simulink model "TSR_Scenario_001_cs"  (R2014b)
settings: Solver=ode5  SolverMode=SingleTasking  StartTime=0.0  StopTime=inf  FixedStep=1/100  RelTol=1e-3
PreLoadFcn:
  | mbxruntime.callbacks.PreLoadFcn(bdroot);
  | check_NUTS_defined;
  | 
  | assignin('base',['model_closed_' bdroot],false);
  | 
  | addpath('../includes_TSR/includes_TSR');
  | 
  | switch version('-release')
  | case {'2010a', '2010b', '2011a'}
  | addpath('../includes_TSR/ML2010b');
  | otherwise
  | addpath('../includes_TSR/ML2011b');
  | end
PostLoadFcn:
  | mbxruntime.callbacks.PostLoadFcn(bdroot);
InitFcn:
  | mbxruntime.callbacks.InitFcn(bdroot);
StartFcn:
  | mbxruntime.callbacks.StartFcn(bdroot);
StopFcn:
  | mbxruntime.callbacks.StopFcn(bdroot);
model workspace: external: MAT-File .\TSR_Scenario_001_cs_hws.mat (data not in the file)
undefined symbols (not defined in the file or in its folder): InitImageOutputDir, mbxruntime, OrientationPitch, OrientationRoll, PositionX, PositionY, PositionZ, tabledata, warningInitialVelocity, x0
undefined symbols (not defined in the file): SteeringColumn, SteeringWheel, TSR_Scenario_001_cs_0469e6db089af631, TSR_Scenario_001_cs_0511100212e7bc8e, TSR_Scenario_001_cs_0e7e9ae969427aac, TSR_Scenario_001_cs_1093386e49c2fe1f, TSR_Scenario_001_cs_112063adae8cf595, TSR_Scenario_001_cs_20f00d93cd5331c2, TSR_Scenario_001_cs_23e3512474fbfadc, TSR_Scenario_001_cs_366523e1554c6bf4, TSR_Scenario_001_cs_37bce4982c67337a, TSR_Scenario_001_cs_44e6164a5df50f45, TSR_Scenario_001_cs_4963ce12e7ff3247, TSR_Scenario_001_cs_4b3e01fa729ce73a, TSR_Scenario_001_cs_519c34727ce9f069, TSR_Scenario_001_cs_5b66ab60038399a1, TSR_Scenario_001_cs_5baa165dfa1afdcb, TSR_Scenario_001_cs_5f993ce39fa6372c, TSR_Scenario_001_cs_613fdf28e3ff7437, TSR_Scenario_001_cs_67b1406af835d622, TSR_Scenario_001_cs_6ad990c290286b94, TSR_Scenario_001_cs_6c412b69295984e1, TSR_Scenario_001_cs_6d4c0c06b1585ef3, TSR_Scenario_001_cs_6dd019d071bf1235, TSR_Scenario_001_cs_6e9f5883f1a78533, TSR_Scenario_001_cs_80f7223d9ac35404, TSR_Scenario_001_cs_8562b82d3c89ae57, TSR_Scenario_001_cs_8a3a0181ab0babfe, TSR_Scenario_001_cs_8c997348ce80deaf, TSR_Scenario_001_cs_925bd6a073d9fe25, TSR_Scenario_001_cs_961436216add6114, TSR_Scenario_001_cs_991a7959256b2c84, TSR_Scenario_001_cs_9a95ce2c2e753616, TSR_Scenario_001_cs_a98aa9562e8552a9, TSR_Scenario_001_cs_ab44ae81dbfb58cd, TSR_Scenario_001_cs_Actros_2541_2_Path_pathUniqueID, TSR_Scenario_001_cs_ae74836ade6bff5a, TSR_Scenario_001_cs_Audi_A8_1_Dynamics_Simple_initialPitch, TSR_Scenario_001_cs_Audi_A8_1_Dynamics_Simple_initialRoll, TSR_Scenario_001_cs_Audi_A8_1_Dynamics_Simple_initialX, TSR_Scenario_001_cs_Audi_A8_1_Dynamics_Simple_initialY, TSR_Scenario_001_cs_Audi_A8_1_Dynamics_Simple_initialYaw, TSR_Scenario_001_cs_Audi_A8_1_Dynamics_Simple_initialZ, TSR_Scenario_001_cs_Audi_A8_2_Path_pathUniqueID, TSR_Scenario_001_cs_Audi_A8_2_SpeedProfile_speedProfileUniqueID, TSR_Scenario_001_cs_b2eca4eb2fce349a, TSR_Scenario_001_cs_b7bac209c1f2549f, TSR_Scenario_001_cs_bf3dccb66d3255a4, TSR_Scenario_001_cs_bf4c1a5315e3f716, TSR_Scenario_001_cs_BMW_Z3_1_Path_pathUniqueID, TSR_Scenario_001_cs_BMW_Z3_1_SpeedProfile_speedProfileUniqueID, TSR_Scenario_001_cs_BMW_Z3_2_Path_pathUniqueID, TSR_Scenario_001_cs_BMW_Z3_2_SpeedProfile_speedProfileUniqueID, TSR_Scenario_001_cs_c4c8fc4bdece03a9, TSR_Scenario_001_cs_c964c86aa54ad92e, TSR_Scenario_001_cs_cb64d1ef85329755, TSR_Scenario_001_cs_Citroen_C3_1_Path_pathUniqueID, TSR_Scenario_001_cs_Citroen_C3_2_Path_pathUniqueID, TSR_Scenario_001_cs_Citroen_C3_3_Path_pathUniqueID, TSR_Scenario_001_cs_Citroen_C3_4_Path_pathUniqueID ... (+25)
libraries: simulink x21, PreScanSimulinkLibrary x17, simulink_extras x13
(part 3 of 30)

== system TSR_Scenario_001_cs/Audi_A8_1_Indicator_front_right ==
  Audi_A8_1_Indicator_front_right : Inport  Tag=inport/IndicatorFR  OutDataTypeStr=Bus: PRESCAN_VISULIGHTACTUATOR_DATA  SampleTime=1/100  BusOutputAsStruct=on
  Actuator : S-Function  FunctionName=sfun_VisuLightActuator  Parameters=mbxruntime.parameters.convert(UniqueID), mbxruntime.parameters.convert(LightName), mbxruntime.parameters.convert(PivotName), mbxruntime.parameters.convert(TextureResources), mbxruntime.parameters.convert(ColorsObjectName), mbxruntime.parameters.convert(MeshOnColor), mbxruntime.parameters.convert(MeshOffColor),tabledata, TimeStep  EnableBusSupport=off  mask(PreScan Sink Block: VisuActiveLight){UniqueID=253, LightName=Audi_A8_1.LightActuator_8_IndicatorFR_ActiveLight, PivotName=Audi_A8_1.IndicatorFR_pivot, TextureResources={ '14' 'LightMap\GeneralLight.png'}, ColorsObjectName=Audi_A8_1.IndicatorFR, MeshOnColor=[255  165    0    0  255  165    0    0  102  102  102  255  510  420  178  255], MeshOffColor=[255  165    0    0  255  165    0    0  102  102  102  255    0    0    0  255], TimeStep=1/100}
      mask prompts: UniqueID "Parent Unique Identifier"; LightName "Light"; PivotName "Pivot"; TextureResources "Texture Resources"; ColorsObjectName "Light Fixture Color Object"; MeshOnColor "Light Fixture On Color"; MeshOffColor "Light Fixture Off Color"; TimeStep "Simulink time step"
      mask help:
      | The VisuActiveLight block provides a way for detailed animation of Light Sources, such as the indicator, brake, fog and main lights of a vehicle, or a light post.
      |
      | For more information, please click Help.
      mask init:
      | [tabledata] = mbxruntime.parameters.table(UniqueID,LightName,PivotName,TextureResources,ColorsObjectName,MeshOnColor,MeshOffColor);
      mask Help: eval('openHelp(209)')
      mask Display: image(imread('HeadLight.png'))
  wires:
  Audi_A8_1_Indicator_front_right/1 -> Actuator/1

== system TSR_Scenario_001_cs/Audi_A8_1_Indicator_rear_left ==
  Audi_A8_1_Indicator_rear_left : Inport  Tag=inport/IndicatorRL  OutDataTypeStr=Bus: PRESCAN_VISULIGHTACTUATOR_DATA  SampleTime=1/100  BusOutputAsStruct=on
  Actuator : S-Function  FunctionName=sfun_VisuLightActuator  Parameters=mbxruntime.parameters.convert(UniqueID), mbxruntime.parameters.convert(LightName), mbxruntime.parameters.convert(PivotName), mbxruntime.parameters.convert(TextureResources), mbxruntime.parameters.convert(ColorsObjectName), mbxruntime.parameters.convert(MeshOnColor), mbxruntime.parameters.convert(MeshOffColor),tabledata, TimeStep  EnableBusSupport=off  mask(PreScan Sink Block: VisuActiveLight){UniqueID=253, LightName=Audi_A8_1.LightActuator_7_IndicatorRL_ActiveLight, PivotName=Audi_A8_1.IndicatorRL_pivot, TextureResources={ '14' 'LightMap\GeneralLight.png'}, ColorsObjectName=Audi_A8_1.IndicatorRL, MeshOnColor=[255  165    0    0  255  165    0    0  102  102  102  255  510  420  178  255], MeshOffColor=[255  165    0    0  255  165    0    0  102  102  102  255    0    0    0  255], TimeStep=1/100}
      mask prompts: UniqueID "Parent Unique Identifier"; LightName "Light"; PivotName "Pivot"; TextureResources "Texture Resources"; ColorsObjectName "Light Fixture Color Object"; MeshOnColor "Light Fixture On Color"; MeshOffColor "Light Fixture Off Color"; TimeStep "Simulink time step"
      mask help:
      | The VisuActiveLight block provides a way for detailed animation of Light Sources, such as the indicator, brake, fog and main lights of a vehicle, or a light post.
      |
      | For more information, please click Help.
      mask init:
      | [tabledata] = mbxruntime.parameters.table(UniqueID,LightName,PivotName,TextureResources,ColorsObjectName,MeshOnColor,MeshOffColor);
      mask Help: eval('openHelp(209)')
      mask Display: image(imread('HeadLight.png'))
  wires:
  Audi_A8_1_Indicator_rear_left/1 -> Actuator/1

== system TSR_Scenario_001_cs/Audi_A8_1_Indicator_rear_right ==
  Audi_A8_1_Indicator_rear_right : Inport  Tag=inport/IndicatorRR  OutDataTypeStr=Bus: PRESCAN_VISULIGHTACTUATOR_DATA  SampleTime=1/100  BusOutputAsStruct=on
  Actuator : S-Function  FunctionName=sfun_VisuLightActuator  Parameters=mbxruntime.parameters.convert(UniqueID), mbxruntime.parameters.convert(LightName), mbxruntime.parameters.convert(PivotName), mbxruntime.parameters.convert(TextureResources), mbxruntime.parameters.convert(ColorsObjectName), mbxruntime.parameters.convert(MeshOnColor), mbxruntime.parameters.convert(MeshOffColor),tabledata, TimeStep  EnableBusSupport=off  mask(PreScan Sink Block: VisuActiveLight){UniqueID=253, LightName=Audi_A8_1.LightActuator_9_IndicatorRR_ActiveLight, PivotName=Audi_A8_1.IndicatorRR_pivot, TextureResources={ '14' 'LightMap\GeneralLight.png'}, ColorsObjectName=Audi_A8_1.IndicatorRR, MeshOnColor=[255  165    0    0  255  165    0    0  102  102  102  255  510  420  178  255], MeshOffColor=[255  165    0    0  255  165    0    0  102  102  102  255    0    0    0  255], TimeStep=1/100}
      mask prompts: UniqueID "Parent Unique Identifier"; LightName "Light"; PivotName "Pivot"; TextureResources "Texture Resources"; ColorsObjectName "Light Fixture Color Object"; MeshOnColor "Light Fixture On Color"; MeshOffColor "Light Fixture Off Color"; TimeStep "Simulink time step"
      mask help:
      | The VisuActiveLight block provides a way for detailed animation of Light Sources, such as the indicator, brake, fog and main lights of a vehicle, or a light post.
      |
      | For more information, please click Help.
      mask init:
      | [tabledata] = mbxruntime.parameters.table(UniqueID,LightName,PivotName,TextureResources,ColorsObjectName,MeshOnColor,MeshOffColor);
      mask Help: eval('openHelp(209)')
      mask Display: image(imread('HeadLight.png'))
  wires:
  Audi_A8_1_Indicator_rear_right/1 -> Actuator/1

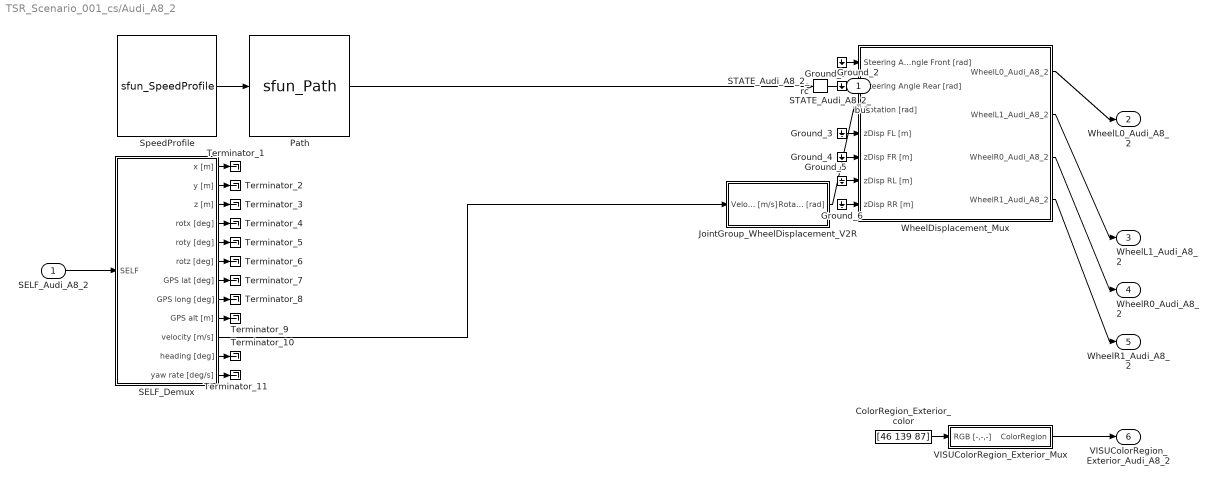
== system TSR_Scenario_001_cs/Audi_A8_2 ==
  SELF_Audi_A8_2 : Inport  Tag=inport/SelfPort  OutDataTypeStr=Bus: PRESCAN_SELFSENSORDATA  PortDimensions=1  SampleTime=1/100  BusOutputAsStruct=on
  ColorRegion_Exterior_color : Constant  Tag=VisuLightConst  Value=[46 139 87]
  Ground_{1..6} (6 alike) : Ground
  JointGroup_WheelDisplacement_V2R : Subsystem  Tag=mux/Wheels  mask(PreScan Velocity to Wheel Angle Block:){TimeStep=1/100, TireRadius=0.29}
      mask prompts: TimeStep "Auto Assigned: Time Step [s]"; TireRadius "Tire Radius [m]"
      settings: DeleteFcn=PreScanBlockDeleteFcn;
      mask Display: disp('Velocity\nto\nWheelAngle')
  Path : S-Function  Tag=Path  LoadFcn=load('PrescanMotionData.mat')  FunctionName=sfun_Path  Parameters=uniqueID, pathUniqueID, timestep  EnableBusSupport=off  mask(Path){uniqueID=1951, pathUniqueID=TSR_Scenario_001_cs_Audi_A8_2_Path_pathUniqueID, timestep=1/100}
      mask prompts: uniqueID "Object Unique ID"; pathUniqueID "Path Unique ID"; timestep "MATLAB timestep:"
      mask help:
      | The path block outputs the position along a given trajectory.
      |
      | For more information, please click Help.
      mask Help: eval('openHelp(312)')
      mask Display: image(imread('Path.png'))
  SELF_Demux : Subsystem  Tag=demux/SelfPort  mask(PreScan Demux Block:){}
      mask help:
      | The SELF port shows (state) information of the actor itself. The outputs are position in the experiment's axis system and the GPS coordinates, and the object's absolute velocity and compass heading.
      |
      | For more information, please click Help.
      settings: DeleteFcn=PreScanBlockDeleteFcn;
      mask Help: eval('openHelp(462)')
      mask Display:
      | port_label('output',1,'x [m]')
      | port_label('output',2,'y [m]')
      | port_label('output',3,'z [m]','texmode','on')
      | port_label('output',4,'Rotx [deg]','texmode','on')
      | port_label('output',5,'Roty [deg]','texmode','on')
      | port_label('output',6,'Rotz [deg]','texmode','on')
      | port_label('output',7,'GPS lat [deg]','texmode','on')
      | port_label('output',8,'GPS long [deg]','texmode','on')
      | port_label('output',9,'GPS alt [m]','texmode','on')
      | port_label('output',10,'Velocity [m/s]')
      | port_label('output',11,'Heading [deg]')
      | port_label('output',12,'Yaw rate [deg/s]')
  STATE_Audi_A8_2_rc : RateTransition  Tag=mux_rc/StatePort  OutPortSampleTimeOpt=Inherit
  SpeedProfile : S-Function  Tag=SpeedProfile  LoadFcn=load('PrescanMotionData.mat')  FunctionName=sfun_SpeedProfile  Parameters=speedProfileUniqueID, timestep  EnableBusSupport=off  mask(SpeedProfile){speedProfileUniqueID=TSR_Scenario_001_cs_Audi_A8_2_SpeedProfile_speedProfileUniqueID, timestep=1/100}
      mask prompts: speedProfileUniqueID "Speed Profile Unique ID"; timestep "MATLAB timestep:"
      mask help:
      | The speed profile block outputs the travelled distance, velocities and acceleration along a given path.
      |
      | For more information, please click Help.
      mask Help: eval('openHelp(312)')
      mask Display: image(imread('SpeedProfile.png'))
  Terminator_{1..11} (11 alike) : Terminator
  VISUColorRegion_Exterior_Mux : Subsystem  Tag=mux/MuxColorRegion  LoadFcn=load PrescanColorData  mask(PreScan User Interface: VisuTextureColor){}
      mask help:
      | The VisuTextureColor block provides a way to adapt the color of a vehicle.
      |
      | For more information, please click Help.
      settings: DeleteFcn=PreScanBlockDeleteFcn;
      mask Help: eval('openHelp(230)')
  WheelDisplacement_Mux : Subsystem  Tag=mux/JointGroup  mask(JointGroup){}
      mask help:
      | The JointGroup allows to control several Joints in one go, as defined for this particular model.
      | For more information, look in the PreScan manual in the section "Model Preparation Tool" -> "Joint Groups"
      |
      | For more information on the Joints simulink interface, press Help.
      mask Help: eval('openHelp(254)')
  STATE_Audi_A8_2_bus : Outport  Tag=outport/StatePort  OutDataTypeStr=Bus: PRESCAN_STATEACTUATORDATA  PortDimensions=1  SampleTime=1/100
  WheelL0_Audi_A8_2 : Outport  Tag=outport/JointActuator  Port=2  OutDataTypeStr=Bus: PRESCAN_POSE_DATA  SampleTime=1/100
  WheelL1_Audi_A8_2 : Outport  Tag=outport/JointActuator  Port=3  OutDataTypeStr=Bus: PRESCAN_POSE_DATA  SampleTime=1/100
  WheelR0_Audi_A8_2 : Outport  Tag=outport/JointActuator  Port=4  OutDataTypeStr=Bus: PRESCAN_POSE_DATA  SampleTime=1/100
  WheelR1_Audi_A8_2 : Outport  Tag=outport/JointActuator  Port=5  OutDataTypeStr=Bus: PRESCAN_POSE_DATA  SampleTime=1/100
  VISUColorRegion_Exterior_Audi_A8_2 : Outport  Tag=outport/ColorRegion  Port=6  OutDataTypeStr=Bus: PRESCAN_COLOR_DATA  PortDimensions=1  SampleTime=1/100
  wires:
  SELF_Demux/10(velocity [m/s]) -> JointGroup_WheelDisplacement_V2R/1(Velocity [m/s])
  STATE_Audi_A8_2_rc/1 -> STATE_Audi_A8_2_bus/1
  SpeedProfile/1 -> Path/1
  Path/1 -> STATE_Audi_A8_2_rc/1
  SELF_Audi_A8_2/1 -> SELF_Demux/1(SELF)
  WheelDisplacement_Mux/1(WheelL0_Audi_A8_2) -> WheelL0_Audi_A8_2/1
  WheelDisplacement_Mux/2(WheelL1_Audi_A8_2) -> WheelL1_Audi_A8_2/1
  WheelDisplacement_Mux/3(WheelR0_Audi_A8_2) -> WheelR0_Audi_A8_2/1
  WheelDisplacement_Mux/4(WheelR1_Audi_A8_2) -> WheelR1_Audi_A8_2/1
  JointGroup_WheelDisplacement_V2R/1(Rotation [rad]) -> WheelDisplacement_Mux/3(Rotation [rad])
  VISUColorRegion_Exterior_Mux/1(ColorRegion) -> VISUColorRegion_Exterior_Audi_A8_2/1
  ColorRegion_Exterior_color/1 -> VISUColorRegion_Exterior_Mux/1(RGB [-,-,-])
  SELF_Demux/1(x [m]) -> Terminator_1/1
  SELF_Demux/2(y [m]) -> Terminator_2/1
  SELF_Demux/3(z [m]) -> Terminator_3/1
  SELF_Demux/4(rotx [deg]) -> Terminator_4/1
  SELF_Demux/5(roty [deg]) -> Terminator_5/1
  SELF_Demux/6(rotz [deg]) -> Terminator_6/1
  SELF_Demux/7(GPS lat [deg]) -> Terminator_7/1
  SELF_Demux/8(GPS long [deg]) -> Terminator_8/1
  SELF_Demux/9(GPS alt [m]) -> Terminator_9/1
  SELF_Demux/11(heading [deg]) -> Terminator_10/1
  SELF_Demux/12(yaw rate [deg/s]) -> Terminator_11/1
  Ground_1/1 -> WheelDisplacement_Mux/1(Steering Angle Front [rad])
  Ground_2/1 -> WheelDisplacement_Mux/2(Steering Angle Rear [rad])
  Ground_3/1 -> WheelDisplacement_Mux/4(zDisp FL [m])
  Ground_4/1 -> WheelDisplacement_Mux/5(zDisp FR [m])
  Ground_5/1 -> WheelDisplacement_Mux/6(zDisp RL [m])
  Ground_6/1 -> WheelDisplacement_Mux/7(zDisp RR [m])

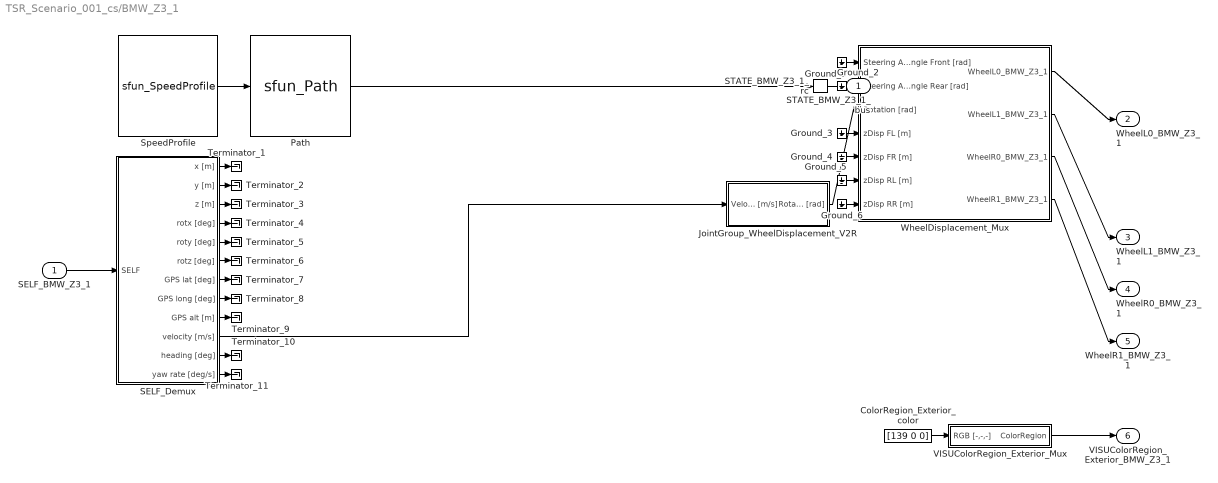
== system TSR_Scenario_001_cs/BMW_Z3_1 ==
  SELF_BMW_Z3_1 : Inport  Tag=inport/SelfPort  OutDataTypeStr=Bus: PRESCAN_SELFSENSORDATA  PortDimensions=1  SampleTime=1/100  BusOutputAsStruct=on
  ColorRegion_Exterior_color : Constant  Tag=VisuLightConst  Value=[139 0 0]
  Ground_{1..6} (6 alike) : Ground
  JointGroup_WheelDisplacement_V2R : Subsystem  Tag=mux/Wheels  mask(PreScan Velocity to Wheel Angle Block:){TimeStep=1/100, TireRadius=0.29}
      mask prompts: TimeStep "Auto Assigned: Time Step [s]"; TireRadius "Tire Radius [m]"
      settings: DeleteFcn=PreScanBlockDeleteFcn;
      mask Display: disp('Velocity\nto\nWheelAngle')
  Path : S-Function  Tag=Path  LoadFcn=load('PrescanMotionData.mat')  FunctionName=sfun_Path  Parameters=uniqueID, pathUniqueID, timestep  EnableBusSupport=off  mask(Path){uniqueID=1948, pathUniqueID=TSR_Scenario_001_cs_BMW_Z3_1_Path_pathUniqueID, timestep=1/100}
      mask prompts: uniqueID "Object Unique ID"; pathUniqueID "Path Unique ID"; timestep "MATLAB timestep:"
      mask help:
      | The path block outputs the position along a given trajectory.
      |
      | For more information, please click Help.
      mask Help: eval('openHelp(312)')
      mask Display: image(imread('Path.png'))
  SELF_Demux : Subsystem  Tag=demux/SelfPort  mask(PreScan Demux Block:){}
      mask help:
      | The SELF port shows (state) information of the actor itself. The outputs are position in the experiment's axis system and the GPS coordinates, and the object's absolute velocity and compass heading.
      |
      | For more information, please click Help.
      settings: DeleteFcn=PreScanBlockDeleteFcn;
      mask Help: eval('openHelp(462)')
      mask Display:
      | port_label('output',1,'x [m]')
      | port_label('output',2,'y [m]')
      | port_label('output',3,'z [m]','texmode','on')
      | port_label('output',4,'Rotx [deg]','texmode','on')
      | port_label('output',5,'Roty [deg]','texmode','on')
      | port_label('output',6,'Rotz [deg]','texmode','on')
      | port_label('output',7,'GPS lat [deg]','texmode','on')
      | port_label('output',8,'GPS long [deg]','texmode','on')
      | port_label('output',9,'GPS alt [m]','texmode','on')
      | port_label('output',10,'Velocity [m/s]')
      | port_label('output',11,'Heading [deg]')
      | port_label('output',12,'Yaw rate [deg/s]')
  STATE_BMW_Z3_1_rc : RateTransition  Tag=mux_rc/StatePort  OutPortSampleTimeOpt=Inherit
  SpeedProfile : S-Function  Tag=SpeedProfile  LoadFcn=load('PrescanMotionData.mat')  FunctionName=sfun_SpeedProfile  Parameters=speedProfileUniqueID, timestep  EnableBusSupport=off  mask(SpeedProfile){speedProfileUniqueID=TSR_Scenario_001_cs_BMW_Z3_1_SpeedProfile_speedProfileUniqueID, timestep=1/100}
      mask prompts: speedProfileUniqueID "Speed Profile Unique ID"; timestep "MATLAB timestep:"
      mask help:
      | The speed profile block outputs the travelled distance, velocities and acceleration along a given path.
      |
      | For more information, please click Help.
      mask Help: eval('openHelp(312)')
      mask Display: image(imread('SpeedProfile.png'))
  Terminator_{1..11} (11 alike) : Terminator
  VISUColorRegion_Exterior_Mux : Subsystem  Tag=mux/MuxColorRegion  LoadFcn=load PrescanColorData  mask(PreScan User Interface: VisuTextureColor){}
      mask help:
      | The VisuTextureColor block provides a way to adapt the color of a vehicle.
      |
      | For more information, please click Help.
      settings: DeleteFcn=PreScanBlockDeleteFcn;
      mask Help: eval('openHelp(230)')
  WheelDisplacement_Mux : Subsystem  Tag=mux/JointGroup  mask(JointGroup){}
      mask help:
      | The JointGroup allows to control several Joints in one go, as defined for this particular model.
      | For more information, look in the PreScan manual in the section "Model Preparation Tool" -> "Joint Groups"
      |
      | For more information on the Joints simulink interface, press Help.
      mask Help: eval('openHelp(254)')
  STATE_BMW_Z3_1_bus : Outport  Tag=outport/StatePort  OutDataTypeStr=Bus: PRESCAN_STATEACTUATORDATA  PortDimensions=1  SampleTime=1/100
  WheelL0_BMW_Z3_1 : Outport  Tag=outport/JointActuator  Port=2  OutDataTypeStr=Bus: PRESCAN_POSE_DATA  SampleTime=1/100
  WheelL1_BMW_Z3_1 : Outport  Tag=outport/JointActuator  Port=3  OutDataTypeStr=Bus: PRESCAN_POSE_DATA  SampleTime=1/100
  WheelR0_BMW_Z3_1 : Outport  Tag=outport/JointActuator  Port=4  OutDataTypeStr=Bus: PRESCAN_POSE_DATA  SampleTime=1/100
  WheelR1_BMW_Z3_1 : Outport  Tag=outport/JointActuator  Port=5  OutDataTypeStr=Bus: PRESCAN_POSE_DATA  SampleTime=1/100
  VISUColorRegion_Exterior_BMW_Z3_1 : Outport  Tag=outport/ColorRegion  Port=6  OutDataTypeStr=Bus: PRESCAN_COLOR_DATA  PortDimensions=1  SampleTime=1/100
  wires:
  SELF_Demux/10(velocity [m/s]) -> JointGroup_WheelDisplacement_V2R/1(Velocity [m/s])
  STATE_BMW_Z3_1_rc/1 -> STATE_BMW_Z3_1_bus/1
  SpeedProfile/1 -> Path/1
  Path/1 -> STATE_BMW_Z3_1_rc/1
  SELF_BMW_Z3_1/1 -> SELF_Demux/1(SELF)
  WheelDisplacement_Mux/1(WheelL0_BMW_Z3_1) -> WheelL0_BMW_Z3_1/1
  WheelDisplacement_Mux/2(WheelL1_BMW_Z3_1) -> WheelL1_BMW_Z3_1/1
  WheelDisplacement_Mux/3(WheelR0_BMW_Z3_1) -> WheelR0_BMW_Z3_1/1
  WheelDisplacement_Mux/4(WheelR1_BMW_Z3_1) -> WheelR1_BMW_Z3_1/1
  JointGroup_WheelDisplacement_V2R/1(Rotation [rad]) -> WheelDisplacement_Mux/3(Rotation [rad])
  VISUColorRegion_Exterior_Mux/1(ColorRegion) -> VISUColorRegion_Exterior_BMW_Z3_1/1
  ColorRegion_Exterior_color/1 -> VISUColorRegion_Exterior_Mux/1(RGB [-,-,-])
  SELF_Demux/1(x [m]) -> Terminator_1/1
  SELF_Demux/2(y [m]) -> Terminator_2/1
  SELF_Demux/3(z [m]) -> Terminator_3/1
  SELF_Demux/4(rotx [deg]) -> Terminator_4/1
  SELF_Demux/5(roty [deg]) -> Terminator_5/1
  SELF_Demux/6(rotz [deg]) -> Terminator_6/1
  SELF_Demux/7(GPS lat [deg]) -> Terminator_7/1
  SELF_Demux/8(GPS long [deg]) -> Terminator_8/1
  SELF_Demux/9(GPS alt [m]) -> Terminator_9/1
  SELF_Demux/11(heading [deg]) -> Terminator_10/1
  SELF_Demux/12(yaw rate [deg/s]) -> Terminator_11/1
  Ground_1/1 -> WheelDisplacement_Mux/1(Steering Angle Front [rad])
  Ground_2/1 -> WheelDisplacement_Mux/2(Steering Angle Rear [rad])
  Ground_3/1 -> WheelDisplacement_Mux/4(zDisp FL [m])
  Ground_4/1 -> WheelDisplacement_Mux/5(zDisp FR [m])
  Ground_5/1 -> WheelDisplacement_Mux/6(zDisp RL [m])
  Ground_6/1 -> WheelDisplacement_Mux/7(zDisp RR [m])

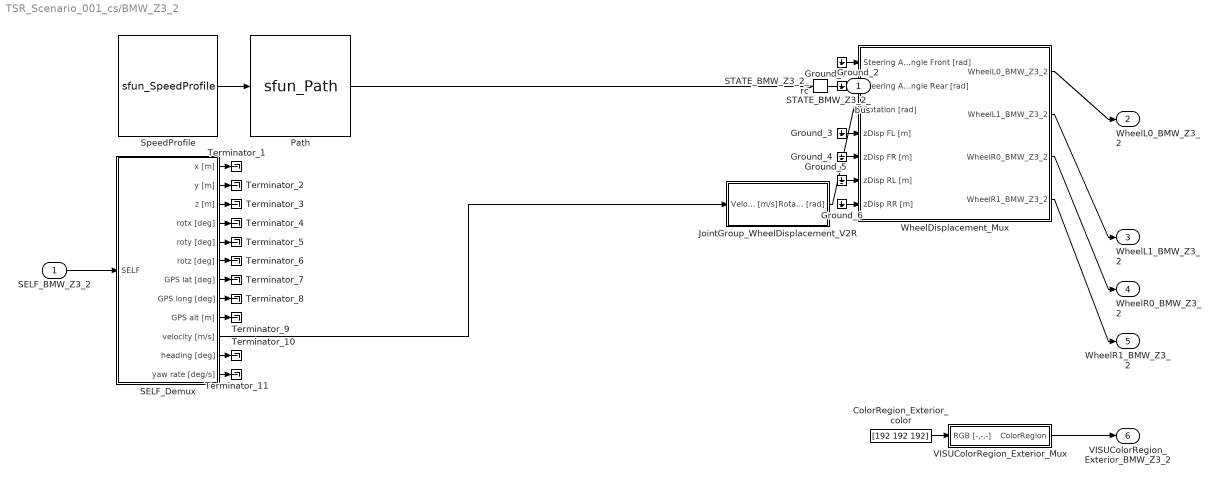
== system TSR_Scenario_001_cs/BMW_Z3_2 ==
  SELF_BMW_Z3_2 : Inport  Tag=inport/SelfPort  OutDataTypeStr=Bus: PRESCAN_SELFSENSORDATA  PortDimensions=1  SampleTime=1/100  BusOutputAsStruct=on
  ColorRegion_Exterior_color : Constant  Tag=VisuLightConst  Value=[192 192 192]
  Ground_{1..6} (6 alike) : Ground
  JointGroup_WheelDisplacement_V2R : Subsystem  Tag=mux/Wheels  mask(PreScan Velocity to Wheel Angle Block:){TimeStep=1/100, TireRadius=0.29}
      mask prompts: TimeStep "Auto Assigned: Time Step [s]"; TireRadius "Tire Radius [m]"
      settings: DeleteFcn=PreScanBlockDeleteFcn;
      mask Display: disp('Velocity\nto\nWheelAngle')
  Path : S-Function  Tag=Path  LoadFcn=load('PrescanMotionData.mat')  FunctionName=sfun_Path  Parameters=uniqueID, pathUniqueID, timestep  EnableBusSupport=off  mask(Path){uniqueID=2024, pathUniqueID=TSR_Scenario_001_cs_BMW_Z3_2_Path_pathUniqueID, timestep=1/100}
      mask prompts: uniqueID "Object Unique ID"; pathUniqueID "Path Unique ID"; timestep "MATLAB timestep:"
      mask help:
      | The path block outputs the position along a given trajectory.
      |
      | For more information, please click Help.
      mask Help: eval('openHelp(312)')
      mask Display: image(imread('Path.png'))
  SELF_Demux : Subsystem  Tag=demux/SelfPort  mask(PreScan Demux Block:){}
      mask help:
      | The SELF port shows (state) information of the actor itself. The outputs are position in the experiment's axis system and the GPS coordinates, and the object's absolute velocity and compass heading.
      |
      | For more information, please click Help.
      settings: DeleteFcn=PreScanBlockDeleteFcn;
      mask Help: eval('openHelp(462)')
      mask Display:
      | port_label('output',1,'x [m]')
      | port_label('output',2,'y [m]')
      | port_label('output',3,'z [m]','texmode','on')
      | port_label('output',4,'Rotx [deg]','texmode','on')
      | port_label('output',5,'Roty [deg]','texmode','on')
      | port_label('output',6,'Rotz [deg]','texmode','on')
      | port_label('output',7,'GPS lat [deg]','texmode','on')
      | port_label('output',8,'GPS long [deg]','texmode','on')
      | port_label('output',9,'GPS alt [m]','texmode','on')
      | port_label('output',10,'Velocity [m/s]')
      | port_label('output',11,'Heading [deg]')
      | port_label('output',12,'Yaw rate [deg/s]')
  STATE_BMW_Z3_2_rc : RateTransition  Tag=mux_rc/StatePort  OutPortSampleTimeOpt=Inherit
  SpeedProfile : S-Function  Tag=SpeedProfile  LoadFcn=load('PrescanMotionData.mat')  FunctionName=sfun_SpeedProfile  Parameters=speedProfileUniqueID, timestep  EnableBusSupport=off  mask(SpeedProfile){speedProfileUniqueID=TSR_Scenario_001_cs_BMW_Z3_2_SpeedProfile_speedProfileUniqueID, timestep=1/100}
      mask prompts: speedProfileUniqueID "Speed Profile Unique ID"; timestep "MATLAB timestep:"
      mask help:
      | The speed profile block outputs the travelled distance, velocities and acceleration along a given path.
      |
      | For more information, please click Help.
      mask Help: eval('openHelp(312)')
      mask Display: image(imread('SpeedProfile.png'))
  Terminator_{1..11} (11 alike) : Terminator
  VISUColorRegion_Exterior_Mux : Subsystem  Tag=mux/MuxColorRegion  LoadFcn=load PrescanColorData  mask(PreScan User Interface: VisuTextureColor){}
      mask help:
      | The VisuTextureColor block provides a way to adapt the color of a vehicle.
      |
      | For more information, please click Help.
      settings: DeleteFcn=PreScanBlockDeleteFcn;
      mask Help: eval('openHelp(230)')
  WheelDisplacement_Mux : Subsystem  Tag=mux/JointGroup  mask(JointGroup){}
      mask help:
      | The JointGroup allows to control several Joints in one go, as defined for this particular model.
      | For more information, look in the PreScan manual in the section "Model Preparation Tool" -> "Joint Groups"
      |
      | For more information on the Joints simulink interface, press Help.
      mask Help: eval('openHelp(254)')
  STATE_BMW_Z3_2_bus : Outport  Tag=outport/StatePort  OutDataTypeStr=Bus: PRESCAN_STATEACTUATORDATA  PortDimensions=1  SampleTime=1/100
  WheelL0_BMW_Z3_2 : Outport  Tag=outport/JointActuator  Port=2  OutDataTypeStr=Bus: PRESCAN_POSE_DATA  SampleTime=1/100
  WheelL1_BMW_Z3_2 : Outport  Tag=outport/JointActuator  Port=3  OutDataTypeStr=Bus: PRESCAN_POSE_DATA  SampleTime=1/100
  WheelR0_BMW_Z3_2 : Outport  Tag=outport/JointActuator  Port=4  OutDataTypeStr=Bus: PRESCAN_POSE_DATA  SampleTime=1/100
  WheelR1_BMW_Z3_2 : Outport  Tag=outport/JointActuator  Port=5  OutDataTypeStr=Bus: PRESCAN_POSE_DATA  SampleTime=1/100
  VISUColorRegion_Exterior_BMW_Z3_2 : Outport  Tag=outport/ColorRegion  Port=6  OutDataTypeStr=Bus: PRESCAN_COLOR_DATA  PortDimensions=1  SampleTime=1/100
  wires:
  SELF_Demux/10(velocity [m/s]) -> JointGroup_WheelDisplacement_V2R/1(Velocity [m/s])
  STATE_BMW_Z3_2_rc/1 -> STATE_BMW_Z3_2_bus/1
  SpeedProfile/1 -> Path/1
  Path/1 -> STATE_BMW_Z3_2_rc/1
  SELF_BMW_Z3_2/1 -> SELF_Demux/1(SELF)
  WheelDisplacement_Mux/1(WheelL0_BMW_Z3_2) -> WheelL0_BMW_Z3_2/1
  WheelDisplacement_Mux/2(WheelL1_BMW_Z3_2) -> WheelL1_BMW_Z3_2/1
  WheelDisplacement_Mux/3(WheelR0_BMW_Z3_2) -> WheelR0_BMW_Z3_2/1
  WheelDisplacement_Mux/4(WheelR1_BMW_Z3_2) -> WheelR1_BMW_Z3_2/1
  JointGroup_WheelDisplacement_V2R/1(Rotation [rad]) -> WheelDisplacement_Mux/3(Rotation [rad])
  VISUColorRegion_Exterior_Mux/1(ColorRegion) -> VISUColorRegion_Exterior_BMW_Z3_2/1
  ColorRegion_Exterior_color/1 -> VISUColorRegion_Exterior_Mux/1(RGB [-,-,-])
  SELF_Demux/1(x [m]) -> Terminator_1/1
  SELF_Demux/2(y [m]) -> Terminator_2/1
  SELF_Demux/3(z [m]) -> Terminator_3/1
  SELF_Demux/4(rotx [deg]) -> Terminator_4/1
  SELF_Demux/5(roty [deg]) -> Terminator_5/1
  SELF_Demux/6(rotz [deg]) -> Terminator_6/1
  SELF_Demux/7(GPS lat [deg]) -> Terminator_7/1
  SELF_Demux/8(GPS long [deg]) -> Terminator_8/1
  SELF_Demux/9(GPS alt [m]) -> Terminator_9/1
  SELF_Demux/11(heading [deg]) -> Terminator_10/1
  SELF_Demux/12(yaw rate [deg/s]) -> Terminator_11/1
  Ground_1/1 -> WheelDisplacement_Mux/1(Steering Angle Front [rad])
  Ground_2/1 -> WheelDisplacement_Mux/2(Steering Angle Rear [rad])
  Ground_3/1 -> WheelDisplacement_Mux/4(zDisp FL [m])
  Ground_4/1 -> WheelDisplacement_Mux/5(zDisp FR [m])
  Ground_5/1 -> WheelDisplacement_Mux/6(zDisp RL [m])
  Ground_6/1 -> WheelDisplacement_Mux/7(zDisp RR [m])

== system TSR_Scenario_001_cs/CameraSensor_1 ==
  Sensor : S-Function  FunctionName=sfun_Camera  Parameters=sensorID, dataWidth, dataHeight, channelsPerImage, numberOfImages, timestep  EnableBusSupport=off  mask(PreScan Source Block: Camera Sensor){sensorID=269, dataWidth=600, dataHeight=2400, channelsPerImage=3, numberOfImages=1, timestep=1/50}
      mask prompts: sensorID "Sensor ID"; dataWidth "Data width"; dataHeight "Data Height"; channelsPerImage "Channels per image"; numberOfImages "Number of images"; timestep "MATLAB timestep:"
      mask help: The Camera Sensor provides a color or monochrome image.
      mask Help: eval('openHelp(457)')
      mask Display: image(imread('CameraSensor.png'))
  CameraSensor_1 : Outport  Tag=outport/Camera/CameraSensor  OutDataTypeStr=uint8  SampleTime=1/50
  wires:
  Sensor/1 -> CameraSensor_1/1

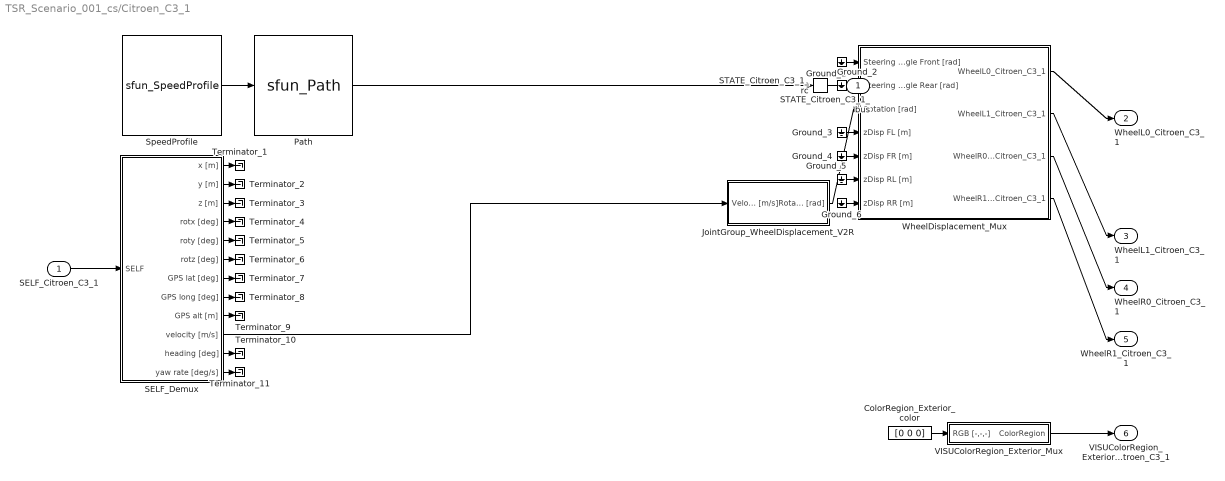
== system TSR_Scenario_001_cs/Citroen_C3_1 ==
  SELF_Citroen_C3_1 : Inport  Tag=inport/SelfPort  OutDataTypeStr=Bus: PRESCAN_SELFSENSORDATA  PortDimensions=1  SampleTime=1/100  BusOutputAsStruct=on
  ColorRegion_Exterior_color : Constant  Tag=VisuLightConst  Value=[0 0 0]
  Ground_{1..6} (6 alike) : Ground
  JointGroup_WheelDisplacement_V2R : Subsystem  Tag=mux/Wheels  mask(PreScan Velocity to Wheel Angle Block:){TimeStep=1/100, TireRadius=0.29}
      mask prompts: TimeStep "Auto Assigned: Time Step [s]"; TireRadius "Tire Radius [m]"
      settings: DeleteFcn=PreScanBlockDeleteFcn;
      mask Display: disp('Velocity\nto\nWheelAngle')
  Path : S-Function  Tag=Path  LoadFcn=load('PrescanMotionData.mat')  FunctionName=sfun_Path  Parameters=uniqueID, pathUniqueID, timestep  EnableBusSupport=off  mask(Path){uniqueID=1955, pathUniqueID=TSR_Scenario_001_cs_Citroen_C3_1_Path_pathUniqueID, timestep=1/100}
      mask prompts: uniqueID "Object Unique ID"; pathUniqueID "Path Unique ID"; timestep "MATLAB timestep:"
      mask help:
      | The path block outputs the position along a given trajectory.
      |
      | For more information, please click Help.
      mask Help: eval('openHelp(312)')
      mask Display: image(imread('Path.png'))
  SELF_Demux : Subsystem  Tag=demux/SelfPort  mask(PreScan Demux Block:){}
      mask help:
      | The SELF port shows (state) information of the actor itself. The outputs are position in the experiment's axis system and the GPS coordinates, and the object's absolute velocity and compass heading.
      |
      | For more information, please click Help.
      settings: DeleteFcn=PreScanBlockDeleteFcn;
      mask Help: eval('openHelp(462)')
      mask Display:
      | port_label('output',1,'x [m]')
      | port_label('output',2,'y [m]')
      | port_label('output',3,'z [m]','texmode','on')
      | port_label('output',4,'Rotx [deg]','texmode','on')
      | port_label('output',5,'Roty [deg]','texmode','on')
      | port_label('output',6,'Rotz [deg]','texmode','on')
      | port_label('output',7,'GPS lat [deg]','texmode','on')
      | port_label('output',8,'GPS long [deg]','texmode','on')
      | port_label('output',9,'GPS alt [m]','texmode','on')
      | port_label('output',10,'Velocity [m/s]')
      | port_label('output',11,'Heading [deg]')
      | port_label('output',12,'Yaw rate [deg/s]')
  STATE_Citroen_C3_1_rc : RateTransition  Tag=mux_rc/StatePort  OutPortSampleTimeOpt=Inherit
  SpeedProfile : S-Function  Tag=SpeedProfile  LoadFcn=load('PrescanMotionData.mat')  FunctionName=sfun_SpeedProfile  Parameters=speedProfileUniqueID, timestep  EnableBusSupport=off  mask(SpeedProfile){speedProfileUniqueID=TSR_Scenario_001_cs_8a3a0181ab0babfe, timestep=1/100}
      mask prompts: speedProfileUniqueID "Speed Profile Unique ID"; timestep "MATLAB timestep:"
      mask help:
      | The speed profile block outputs the travelled distance, velocities and acceleration along a given path.
      |
      | For more information, please click Help.
      mask Help: eval('openHelp(312)')
      mask Display: image(imread('SpeedProfile.png'))
  Terminator_{1..11} (11 alike) : Terminator
  VISUColorRegion_Exterior_Mux : Subsystem  Tag=mux/MuxColorRegion  LoadFcn=load PrescanColorData  mask(PreScan User Interface: VisuTextureColor){}
      mask help:
      | The VisuTextureColor block provides a way to adapt the color of a vehicle.
      |
      | For more information, please click Help.
      settings: DeleteFcn=PreScanBlockDeleteFcn;
      mask Help: eval('openHelp(230)')
  WheelDisplacement_Mux : Subsystem  Tag=mux/JointGroup  mask(JointGroup){}
      mask help:
      | The JointGroup allows to control several Joints in one go, as defined for this particular model.
      | For more information, look in the PreScan manual in the section "Model Preparation Tool" -> "Joint Groups"
      |
      | For more information on the Joints simulink interface, press Help.
      mask Help: eval('openHelp(254)')
  STATE_Citroen_C3_1_bus : Outport  Tag=outport/StatePort  OutDataTypeStr=Bus: PRESCAN_STATEACTUATORDATA  PortDimensions=1  SampleTime=1/100
  WheelL0_Citroen_C3_1 : Outport  Tag=outport/JointActuator  Port=2  OutDataTypeStr=Bus: PRESCAN_POSE_DATA  SampleTime=1/100
  WheelL1_Citroen_C3_1 : Outport  Tag=outport/JointActuator  Port=3  OutDataTypeStr=Bus: PRESCAN_POSE_DATA  SampleTime=1/100
  WheelR0_Citroen_C3_1 : Outport  Tag=outport/JointActuator  Port=4  OutDataTypeStr=Bus: PRESCAN_POSE_DATA  SampleTime=1/100
  WheelR1_Citroen_C3_1 : Outport  Tag=outport/JointActuator  Port=5  OutDataTypeStr=Bus: PRESCAN_POSE_DATA  SampleTime=1/100
  VISUColorRegion_Exterior_Citroen_C3_1 : Outport  Tag=outport/ColorRegion  Port=6  OutDataTypeStr=Bus: PRESCAN_COLOR_DATA  PortDimensions=1  SampleTime=1/100
  wires:
  SELF_Demux/10(velocity [m/s]) -> JointGroup_WheelDisplacement_V2R/1(Velocity [m/s])
  STATE_Citroen_C3_1_rc/1 -> STATE_Citroen_C3_1_bus/1
  SpeedProfile/1 -> Path/1
  Path/1 -> STATE_Citroen_C3_1_rc/1
  SELF_Citroen_C3_1/1 -> SELF_Demux/1(SELF)
  WheelDisplacement_Mux/1(WheelL0_Citroen_C3_1) -> WheelL0_Citroen_C3_1/1
  WheelDisplacement_Mux/2(WheelL1_Citroen_C3_1) -> WheelL1_Citroen_C3_1/1
  WheelDisplacement_Mux/3(WheelR0_Citroen_C3_1) -> WheelR0_Citroen_C3_1/1
  WheelDisplacement_Mux/4(WheelR1_Citroen_C3_1) -> WheelR1_Citroen_C3_1/1
  JointGroup_WheelDisplacement_V2R/1(Rotation [rad]) -> WheelDisplacement_Mux/3(Rotation [rad])
  VISUColorRegion_Exterior_Mux/1(ColorRegion) -> VISUColorRegion_Exterior_Citroen_C3_1/1
  ColorRegion_Exterior_color/1 -> VISUColorRegion_Exterior_Mux/1(RGB [-,-,-])
  SELF_Demux/1(x [m]) -> Terminator_1/1
  SELF_Demux/2(y [m]) -> Terminator_2/1
  SELF_Demux/3(z [m]) -> Terminator_3/1
  SELF_Demux/4(rotx [deg]) -> Terminator_4/1
  SELF_Demux/5(roty [deg]) -> Terminator_5/1
  SELF_Demux/6(rotz [deg]) -> Terminator_6/1
  SELF_Demux/7(GPS lat [deg]) -> Terminator_7/1
  SELF_Demux/8(GPS long [deg]) -> Terminator_8/1
  SELF_Demux/9(GPS alt [m]) -> Terminator_9/1
  SELF_Demux/11(heading [deg]) -> Terminator_10/1
  SELF_Demux/12(yaw rate [deg/s]) -> Terminator_11/1
  Ground_1/1 -> WheelDisplacement_Mux/1(Steering Angle Front [rad])
  Ground_2/1 -> WheelDisplacement_Mux/2(Steering Angle Rear [rad])
  Ground_3/1 -> WheelDisplacement_Mux/4(zDisp FL [m])
  Ground_4/1 -> WheelDisplacement_Mux/5(zDisp FR [m])
  Ground_5/1 -> WheelDisplacement_Mux/6(zDisp RL [m])
  Ground_6/1 -> WheelDisplacement_Mux/7(zDisp RR [m])

== system TSR_Scenario_001_cs/Citroen_C3_2 ==
  SELF_Citroen_C3_2 : Inport  Tag=inport/SelfPort  OutDataTypeStr=Bus: PRESCAN_SELFSENSORDATA  PortDimensions=1  SampleTime=1/100  BusOutputAsStruct=on
  ColorRegion_Exterior_color : Constant  Tag=VisuLightConst  Value=[0 0 255]
  Ground_{1..6} (6 alike) : Ground
  JointGroup_WheelDisplacement_V2R : Subsystem  Tag=mux/Wheels  mask(PreScan Velocity to Wheel Angle Block:){TimeStep=1/100, TireRadius=0.29}
      mask prompts: TimeStep "Auto Assigned: Time Step [s]"; TireRadius "Tire Radius [m]"
      settings: DeleteFcn=PreScanBlockDeleteFcn;
      mask Display: disp('Velocity\nto\nWheelAngle')
  Path : S-Function  Tag=Path  LoadFcn=load('PrescanMotionData.mat')  FunctionName=sfun_Path  Parameters=uniqueID, pathUniqueID, timestep  EnableBusSupport=off  mask(Path){uniqueID=1958, pathUniqueID=TSR_Scenario_001_cs_Citroen_C3_2_Path_pathUniqueID, timestep=1/100}
      mask prompts: uniqueID "Object Unique ID"; pathUniqueID "Path Unique ID"; timestep "MATLAB timestep:"
      mask help:
      | The path block outputs the position along a given trajectory.
      |
      | For more information, please click Help.
      mask Help: eval('openHelp(312)')
      mask Display: image(imread('Path.png'))
  SELF_Demux : Subsystem  Tag=demux/SelfPort  mask(PreScan Demux Block:){}
      mask help:
      | The SELF port shows (state) information of the actor itself. The outputs are position in the experiment's axis system and the GPS coordinates, and the object's absolute velocity and compass heading.
      |
      | For more information, please click Help.
      settings: DeleteFcn=PreScanBlockDeleteFcn;
      mask Help: eval('openHelp(462)')
      mask Display:
      | port_label('output',1,'x [m]')
      | port_label('output',2,'y [m]')
      | port_label('output',3,'z [m]','texmode','on')
      | port_label('output',4,'Rotx [deg]','texmode','on')
      | port_label('output',5,'Roty [deg]','texmode','on')
      | port_label('output',6,'Rotz [deg]','texmode','on')
      | port_label('output',7,'GPS lat [deg]','texmode','on')
      | port_label('output',8,'GPS long [deg]','texmode','on')
      | port_label('output',9,'GPS alt [m]','texmode','on')
      | port_label('output',10,'Velocity [m/s]')
      | port_label('output',11,'Heading [deg]')
      | port_label('output',12,'Yaw rate [deg/s]')
  STATE_Citroen_C3_2_rc : RateTransition  Tag=mux_rc/StatePort  OutPortSampleTimeOpt=Inherit
  SpeedProfile : S-Function  Tag=SpeedProfile  LoadFcn=load('PrescanMotionData.mat')  FunctionName=sfun_SpeedProfile  Parameters=speedProfileUniqueID, timestep  EnableBusSupport=off  mask(SpeedProfile){speedProfileUniqueID=TSR_Scenario_001_cs_0e7e9ae969427aac, timestep=1/100}
      mask prompts: speedProfileUniqueID "Speed Profile Unique ID"; timestep "MATLAB timestep:"
      mask help:
      | The speed profile block outputs the travelled distance, velocities and acceleration along a given path.
      |
      | For more information, please click Help.
      mask Help: eval('openHelp(312)')
      mask Display: image(imread('SpeedProfile.png'))
  Terminator_{1..11} (11 alike) : Terminator
  VISUColorRegion_Exterior_Mux : Subsystem  Tag=mux/MuxColorRegion  LoadFcn=load PrescanColorData  mask(PreScan User Interface: VisuTextureColor){}
      mask help:
      | The VisuTextureColor block provides a way to adapt the color of a vehicle.
      |
      | For more information, please click Help.
      settings: DeleteFcn=PreScanBlockDeleteFcn;
      mask Help: eval('openHelp(230)')
  WheelDisplacement_Mux : Subsystem  Tag=mux/JointGroup  mask(JointGroup){}
      mask help:
      | The JointGroup allows to control several Joints in one go, as defined for this particular model.
      | For more information, look in the PreScan manual in the section "Model Preparation Tool" -> "Joint Groups"
      |
      | For more information on the Joints simulink interface, press Help.
      mask Help: eval('openHelp(254)')
  STATE_Citroen_C3_2_bus : Outport  Tag=outport/StatePort  OutDataTypeStr=Bus: PRESCAN_STATEACTUATORDATA  PortDimensions=1  SampleTime=1/100
  WheelL0_Citroen_C3_2 : Outport  Tag=outport/JointActuator  Port=2  OutDataTypeStr=Bus: PRESCAN_POSE_DATA  SampleTime=1/100
  WheelL1_Citroen_C3_2 : Outport  Tag=outport/JointActuator  Port=3  OutDataTypeStr=Bus: PRESCAN_POSE_DATA  SampleTime=1/100
  WheelR0_Citroen_C3_2 : Outport  Tag=outport/JointActuator  Port=4  OutDataTypeStr=Bus: PRESCAN_POSE_DATA  SampleTime=1/100
  WheelR1_Citroen_C3_2 : Outport  Tag=outport/JointActuator  Port=5  OutDataTypeStr=Bus: PRESCAN_POSE_DATA  SampleTime=1/100
  VISUColorRegion_Exterior_Citroen_C3_2 : Outport  Tag=outport/ColorRegion  Port=6  OutDataTypeStr=Bus: PRESCAN_COLOR_DATA  PortDimensions=1  SampleTime=1/100
  wires:
  SELF_Demux/10(velocity [m/s]) -> JointGroup_WheelDisplacement_V2R/1(Velocity [m/s])
  STATE_Citroen_C3_2_rc/1 -> STATE_Citroen_C3_2_bus/1
  SpeedProfile/1 -> Path/1
  Path/1 -> STATE_Citroen_C3_2_rc/1
  SELF_Citroen_C3_2/1 -> SELF_Demux/1(SELF)
  WheelDisplacement_Mux/1(WheelL0_Citroen_C3_2) -> WheelL0_Citroen_C3_2/1
  WheelDisplacement_Mux/2(WheelL1_Citroen_C3_2) -> WheelL1_Citroen_C3_2/1
  WheelDisplacement_Mux/3(WheelR0_Citroen_C3_2) -> WheelR0_Citroen_C3_2/1
  WheelDisplacement_Mux/4(WheelR1_Citroen_C3_2) -> WheelR1_Citroen_C3_2/1
  JointGroup_WheelDisplacement_V2R/1(Rotation [rad]) -> WheelDisplacement_Mux/3(Rotation [rad])
  VISUColorRegion_Exterior_Mux/1(ColorRegion) -> VISUColorRegion_Exterior_Citroen_C3_2/1
  ColorRegion_Exterior_color/1 -> VISUColorRegion_Exterior_Mux/1(RGB [-,-,-])
  SELF_Demux/1(x [m]) -> Terminator_1/1
  SELF_Demux/2(y [m]) -> Terminator_2/1
  SELF_Demux/3(z [m]) -> Terminator_3/1
  SELF_Demux/4(rotx [deg]) -> Terminator_4/1
  SELF_Demux/5(roty [deg]) -> Terminator_5/1
  SELF_Demux/6(rotz [deg]) -> Terminator_6/1
  SELF_Demux/7(GPS lat [deg]) -> Terminator_7/1
  SELF_Demux/8(GPS long [deg]) -> Terminator_8/1
  SELF_Demux/9(GPS alt [m]) -> Terminator_9/1
  SELF_Demux/11(heading [deg]) -> Terminator_10/1
  SELF_Demux/12(yaw rate [deg/s]) -> Terminator_11/1
  Ground_1/1 -> WheelDisplacement_Mux/1(Steering Angle Front [rad])
  Ground_2/1 -> WheelDisplacement_Mux/2(Steering Angle Rear [rad])
  Ground_3/1 -> WheelDisplacement_Mux/4(zDisp FL [m])
  Ground_4/1 -> WheelDisplacement_Mux/5(zDisp FR [m])
  Ground_5/1 -> WheelDisplacement_Mux/6(zDisp RL [m])
  Ground_6/1 -> WheelDisplacement_Mux/7(zDisp RR [m])

== system TSR_Scenario_001_cs/Citroen_C3_3 ==
  SELF_Citroen_C3_3 : Inport  Tag=inport/SelfPort  OutDataTypeStr=Bus: PRESCAN_SELFSENSORDATA  PortDimensions=1  SampleTime=1/100  BusOutputAsStruct=on
  ColorRegion_Exterior_color : Constant  Tag=VisuLightConst  Value=[0 0 128]
  Ground_{1..6} (6 alike) : Ground
  JointGroup_WheelDisplacement_V2R : Subsystem  Tag=mux/Wheels  mask(PreScan Velocity to Wheel Angle Block:){TimeStep=1/100, TireRadius=0.29}
      mask prompts: TimeStep "Auto Assigned: Time Step [s]"; TireRadius "Tire Radius [m]"
      settings: DeleteFcn=PreScanBlockDeleteFcn;
      mask Display: disp('Velocity\nto\nWheelAngle')
  Path : S-Function  Tag=Path  LoadFcn=load('PrescanMotionData.mat')  FunctionName=sfun_Path  Parameters=uniqueID, pathUniqueID, timestep  EnableBusSupport=off  mask(Path){uniqueID=1967, pathUniqueID=TSR_Scenario_001_cs_Citroen_C3_3_Path_pathUniqueID, timestep=1/100}
      mask prompts: uniqueID "Object Unique ID"; pathUniqueID "Path Unique ID"; timestep "MATLAB timestep:"
      mask help:
      | The path block outputs the position along a given trajectory.
      |
      | For more information, please click Help.
      mask Help: eval('openHelp(312)')
      mask Display: image(imread('Path.png'))
  SELF_Demux : Subsystem  Tag=demux/SelfPort  mask(PreScan Demux Block:){}
      mask help:
      | The SELF port shows (state) information of the actor itself. The outputs are position in the experiment's axis system and the GPS coordinates, and the object's absolute velocity and compass heading.
      |
      | For more information, please click Help.
      settings: DeleteFcn=PreScanBlockDeleteFcn;
      mask Help: eval('openHelp(462)')
      mask Display:
      | port_label('output',1,'x [m]')
      | port_label('output',2,'y [m]')
      | port_label('output',3,'z [m]','texmode','on')
      | port_label('output',4,'Rotx [deg]','texmode','on')
      | port_label('output',5,'Roty [deg]','texmode','on')
      | port_label('output',6,'Rotz [deg]','texmode','on')
      | port_label('output',7,'GPS lat [deg]','texmode','on')
      | port_label('output',8,'GPS long [deg]','texmode','on')
      | port_label('output',9,'GPS alt [m]','texmode','on')
      | port_label('output',10,'Velocity [m/s]')
      | port_label('output',11,'Heading [deg]')
      | port_label('output',12,'Yaw rate [deg/s]')
  STATE_Citroen_C3_3_rc : RateTransition  Tag=mux_rc/StatePort  OutPortSampleTimeOpt=Inherit
  SpeedProfile : S-Function  Tag=SpeedProfile  LoadFcn=load('PrescanMotionData.mat')  FunctionName=sfun_SpeedProfile  Parameters=speedProfileUniqueID, timestep  EnableBusSupport=off  mask(SpeedProfile){speedProfileUniqueID=TSR_Scenario_001_cs_80f7223d9ac35404, timestep=1/100}
      mask prompts: speedProfileUniqueID "Speed Profile Unique ID"; timestep "MATLAB timestep:"
      mask help:
      | The speed profile block outputs the travelled distance, velocities and acceleration along a given path.
      |
      | For more information, please click Help.
      mask Help: eval('openHelp(312)')
      mask Display: image(imread('SpeedProfile.png'))
  Terminator_{1..11} (11 alike) : Terminator
  VISUColorRegion_Exterior_Mux : Subsystem  Tag=mux/MuxColorRegion  LoadFcn=load PrescanColorData  mask(PreScan User Interface: VisuTextureColor){}
      mask help:
      | The VisuTextureColor block provides a way to adapt the color of a vehicle.
      |
      | For more information, please click Help.
      settings: DeleteFcn=PreScanBlockDeleteFcn;
      mask Help: eval('openHelp(230)')
  WheelDisplacement_Mux : Subsystem  Tag=mux/JointGroup  mask(JointGroup){}
      mask help:
      | The JointGroup allows to control several Joints in one go, as defined for this particular model.
      | For more information, look in the PreScan manual in the section "Model Preparation Tool" -> "Joint Groups"
      |
      | For more information on the Joints simulink interface, press Help.
      mask Help: eval('openHelp(254)')
  STATE_Citroen_C3_3_bus : Outport  Tag=outport/StatePort  OutDataTypeStr=Bus: PRESCAN_STATEACTUATORDATA  PortDimensions=1  SampleTime=1/100
  WheelL0_Citroen_C3_3 : Outport  Tag=outport/JointActuator  Port=2  OutDataTypeStr=Bus: PRESCAN_POSE_DATA  SampleTime=1/100
  WheelL1_Citroen_C3_3 : Outport  Tag=outport/JointActuator  Port=3  OutDataTypeStr=Bus: PRESCAN_POSE_DATA  SampleTime=1/100
  WheelR0_Citroen_C3_3 : Outport  Tag=outport/JointActuator  Port=4  OutDataTypeStr=Bus: PRESCAN_POSE_DATA  SampleTime=1/100
  WheelR1_Citroen_C3_3 : Outport  Tag=outport/JointActuator  Port=5  OutDataTypeStr=Bus: PRESCAN_POSE_DATA  SampleTime=1/100
  VISUColorRegion_Exterior_Citroen_C3_3 : Outport  Tag=outport/ColorRegion  Port=6  OutDataTypeStr=Bus: PRESCAN_COLOR_DATA  PortDimensions=1  SampleTime=1/100
  wires:
  SELF_Demux/10(velocity [m/s]) -> JointGroup_WheelDisplacement_V2R/1(Velocity [m/s])
  STATE_Citroen_C3_3_rc/1 -> STATE_Citroen_C3_3_bus/1
  SpeedProfile/1 -> Path/1
  Path/1 -> STATE_Citroen_C3_3_rc/1
  SELF_Citroen_C3_3/1 -> SELF_Demux/1(SELF)
  WheelDisplacement_Mux/1(WheelL0_Citroen_C3_3) -> WheelL0_Citroen_C3_3/1
  WheelDisplacement_Mux/2(WheelL1_Citroen_C3_3) -> WheelL1_Citroen_C3_3/1
  WheelDisplacement_Mux/3(WheelR0_Citroen_C3_3) -> WheelR0_Citroen_C3_3/1
  WheelDisplacement_Mux/4(WheelR1_Citroen_C3_3) -> WheelR1_Citroen_C3_3/1
  JointGroup_WheelDisplacement_V2R/1(Rotation [rad]) -> WheelDisplacement_Mux/3(Rotation [rad])
  VISUColorRegion_Exterior_Mux/1(ColorRegion) -> VISUColorRegion_Exterior_Citroen_C3_3/1
  ColorRegion_Exterior_color/1 -> VISUColorRegion_Exterior_Mux/1(RGB [-,-,-])
  SELF_Demux/1(x [m]) -> Terminator_1/1
  SELF_Demux/2(y [m]) -> Terminator_2/1
  SELF_Demux/3(z [m]) -> Terminator_3/1
  SELF_Demux/4(rotx [deg]) -> Terminator_4/1
  SELF_Demux/5(roty [deg]) -> Terminator_5/1
  SELF_Demux/6(rotz [deg]) -> Terminator_6/1
  SELF_Demux/7(GPS lat [deg]) -> Terminator_7/1
  SELF_Demux/8(GPS long [deg]) -> Terminator_8/1
  SELF_Demux/9(GPS alt [m]) -> Terminator_9/1
  SELF_Demux/11(heading [deg]) -> Terminator_10/1
  SELF_Demux/12(yaw rate [deg/s]) -> Terminator_11/1
  Ground_1/1 -> WheelDisplacement_Mux/1(Steering Angle Front [rad])
  Ground_2/1 -> WheelDisplacement_Mux/2(Steering Angle Rear [rad])
  Ground_3/1 -> WheelDisplacement_Mux/4(zDisp FL [m])
  Ground_4/1 -> WheelDisplacement_Mux/5(zDisp FR [m])
  Ground_5/1 -> WheelDisplacement_Mux/6(zDisp RL [m])
  Ground_6/1 -> WheelDisplacement_Mux/7(zDisp RR [m])
